simulink model "matlabVPC"  (R2021a)
settings: Solver=FixedStepAuto  StartTime=0.0  StopTime=tend  FixedStep=0.02  RelTol=1e-3
undefined symbols (not defined in the file): alpha, eta1, eta2, gd, Kc, offset1, offset2, pwo_init, scale1, scale2, T, v1, v2, var_max
libraries: simlib_vpc_basic x17, simlib_vpc_coremath x10, simlib_vpc_gp x3
settings Model: Creator=marco  LastModifiedBy=marco
settings DebuggingCC: AlgebraicLoopMsg=none  ArtificialAlgebraicLoopMsg=none

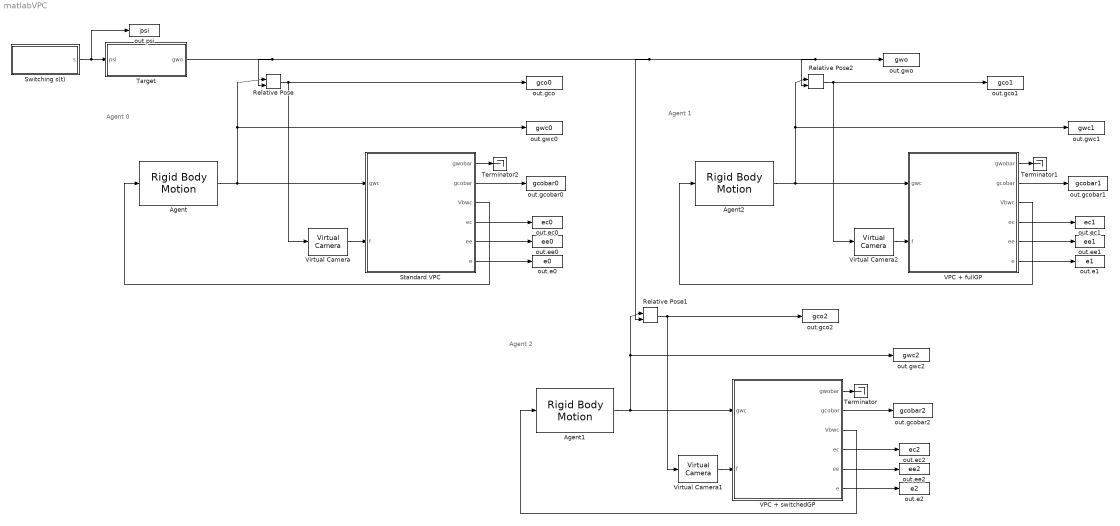
== system matlabVPC ==
  note: Agent 2
  note: Agent 1
  note: Agent 0
  Agent : simlib_vpc_basic/Rigid Body Motion  rbmtype=agent  agentnumber=1  projection=on  show_dg=off  g0=gwc_init
      settings: SourceProductName=VPC Library
  Agent1 : simlib_vpc_basic/Rigid Body Motion  rbmtype=agent  agentnumber=3  projection=on  show_dg=off  g0=gwc_init
      settings: SourceProductName=VPC Library
  Agent2 : simlib_vpc_basic/Rigid Body Motion  rbmtype=agent  agentnumber=2  projection=on  show_dg=off  g0=gwc_init
      settings: SourceProductName=VPC Library
  Relative Pose : simlib_vpc_coremath/Relative Pose
      settings: SourceProductName=VPC Library
  Relative Pose1 : simlib_vpc_coremath/Relative Pose
      settings: SourceProductName=VPC Library
  Relative Pose2 : simlib_vpc_coremath/Relative Pose
      settings: SourceProductName=VPC Library
  Standard VPC : Subsystem
      mask Display:
      | disp('VPC without GP','texmode','on')
      | 
      | % Label ports
      | port_label('input',1,'g_{wc}','texmode','on')
      | port_label('input',2,'f','texmode','on')
      | port_label('output',1,'g_{wo,bar}','texmode','on')
      | port_label('output',2,'gco,bar','texmode','on')
      | port_label('output',3,'V^b_{wc}','texmode','on')
      | port_label('output',4,'ec','texmode','on')
      | port_label('output',5,'ee','texmode','on')
      | port_label('output',6,'e','texmode','on')
  Switching s(t) : Subsystem
  Target : Subsystem
      mask Display:
      | % Glitch in Matlab: If you define a line whose starting point and end point
      | % is equal, then the entire mask block is plotted in bold
      | plot([0,0],[0,0])
      | 
      | % Draw Box
      | plot([0,1,1,0,0],[0,0,1,1,0])
      | 
      | % Write label
      | disp('Target','texmode','on')
      | 
      | % Image
      | p=get_param(gcb,'Position');
      | size = min(p(3:4)-p(1:2));
      | blkscale = abs((p(3)-p(1)) / (p(4)-p(2)));
      | if abs((p(3)-p(1))) > abs((p(4)-p(2))) % block is horizontal
      |     scale = .5*[1/blkscale .6];
      | else % block is vertical
      |     scale = .5*[1 .6*blkscale];
      | end
      | pos = [1-scale(1) 0.1]/2;
      | image('ico_target.png',[pos scale],'off')
      | 
      | % Label ports
      | port_label('output',1,['g_{wo}'],'texmode','on')
  Terminator : Terminator
  Terminator1 : Terminator
  Terminator2 : Terminator
  VPC + fullGP : Subsystem
      mask Display:
      | disp('VPC + fullGP','texmode','on')
      | 
      | % Label ports
      | port_label('input',1,'g_{wc}','texmode','on')
      | port_label('input',2,'f','texmode','on')
      | port_label('output',1,'g_{wo,bar}','texmode','on')
      | port_label('output',2,'gco,bar','texmode','on')
      | port_label('output',3,'V^b_{wc}','texmode','on')
      | port_label('output',4,'ec','texmode','on')
      | port_label('output',5,'ee','texmode','on')
      | port_label('output',6,'e','texmode','on')
  VPC + switchedGP : Subsystem
      mask Display:
      | disp('VPC + switchedGP','texmode','on')
      | 
      | % Label ports
      | port_label('input',1,'g_{wc}','texmode','on')
      | port_label('input',2,'f','texmode','on')
      | port_label('output',1,'g_{wo,bar}','texmode','on')
      | port_label('output',2,'gco,bar','texmode','on')
      | port_label('output',3,'V^b_{wc}','texmode','on')
      | port_label('output',4,'ec','texmode','on')
      | port_label('output',5,'ee','texmode','on')
      | port_label('output',6,'e','texmode','on')
  Virtual Camera : simlib_vpc_basic/Virtual Camera  camtype=Pinhole  po=fp  lambda=lambda
      settings: SourceProductName=VPC Library
  Virtual Camera1 : simlib_vpc_basic/Virtual Camera  camtype=Pinhole  po=fp  lambda=lambda
      settings: SourceProductName=VPC Library
  Virtual Camera2 : simlib_vpc_basic/Virtual Camera  camtype=Pinhole  po=fp  lambda=lambda
      settings: SourceProductName=VPC Library
  out.e0 : ToWorkspace  VariableName=e0  SaveFormat=Structure With Time  SampleTime=-1
  out.e1 : ToWorkspace  VariableName=e1  SaveFormat=Structure With Time  SampleTime=-1
  out.e2 : ToWorkspace  VariableName=e2  SaveFormat=Structure With Time  SampleTime=-1
  out.ec0 : ToWorkspace  VariableName=ec0  SaveFormat=Structure With Time  SampleTime=-1
  out.ec1 : ToWorkspace  VariableName=ec1  SaveFormat=Structure With Time  SampleTime=-1
  out.ec2 : ToWorkspace  VariableName=ec2  SaveFormat=Structure With Time  SampleTime=-1
  out.ee0 : ToWorkspace  VariableName=ee0  SaveFormat=Structure With Time  SampleTime=-1
  out.ee1 : ToWorkspace  VariableName=ee1  SaveFormat=Structure With Time  SampleTime=-1
  out.ee2 : ToWorkspace  VariableName=ee2  SaveFormat=Structure With Time  SampleTime=-1
  out.gco : ToWorkspace  VariableName=gco0  SaveFormat=Structure With Time  SampleTime=-1
  out.gco1 : ToWorkspace  VariableName=gco1  SaveFormat=Structure With Time  SampleTime=-1
  out.gco2 : ToWorkspace  VariableName=gco2  SaveFormat=Structure With Time  SampleTime=-1
  out.gcobar0 : ToWorkspace  VariableName=gcobar0  SaveFormat=Structure With Time  SampleTime=-1
  out.gcobar1 : ToWorkspace  VariableName=gcobar1  SaveFormat=Structure With Time  SampleTime=-1
  out.gcobar2 : ToWorkspace  VariableName=gcobar2  SaveFormat=Structure With Time  SampleTime=-1
  out.gwc0 : ToWorkspace  VariableName=gwc0  SaveFormat=Structure With Time  SampleTime=-1
  out.gwc1 : ToWorkspace  VariableName=gwc1  SaveFormat=Structure With Time  SampleTime=-1
  out.gwc2 : ToWorkspace  VariableName=gwc2  SaveFormat=Structure With Time  SampleTime=-1
  out.gwo : ToWorkspace  VariableName=gwo  SaveFormat=Structure With Time  SampleTime=-1
  out.psi : ToWorkspace  VariableName=psi  SaveFormat=Structure With Time  SampleTime=-1
  wires:
  Relative Pose2/1 -> Virtual Camera2/1, out.gco1/1
  Relative Pose/1 -> Virtual Camera/1, out.gco/1
  VPC + fullGP/2(gcobar) -> out.gcobar1/1
  VPC + switchedGP/4(ec) -> out.ec2/1
  Relative Pose1/1 -> Virtual Camera1/1, out.gco2/1
  Agent1/1 -> VPC + switchedGP/1(gwc), out.gwc2/1, Relative Pose1/1
  Switching s(t)/1(s) -> out.psi/1, Target/1(psi)
  Virtual Camera/1 -> Standard VPC/2(f)
  VPC + switchedGP/2(gcobar) -> out.gcobar2/1
  Virtual Camera2/1 -> VPC + fullGP/2(f)
  VPC + switchedGP/5(ee) -> out.ee2/1
  VPC + fullGP/4(ec) -> out.ec1/1
  VPC + switchedGP/6(e) -> out.e2/1
  Virtual Camera1/1 -> VPC + switchedGP/2(f)
  Agent/1 -> Standard VPC/1(gwc), out.gwc0/1, Relative Pose/1
  Standard VPC/6(e) -> out.e0/1
  Target/1(gwo) -> Relative Pose2/2, out.gwo/1, Relative Pose1/2, Relative Pose/2
  Standard VPC/4(ec) -> out.ec0/1
  Standard VPC/5(ee) -> out.ee0/1
  Agent2/1 -> VPC + fullGP/1(gwc), out.gwc1/1, Relative Pose2/1
  Standard VPC/2(gcobar) -> out.gcobar0/1
  VPC + fullGP/5(ee) -> out.ee1/1
  VPC + fullGP/6(e) -> out.e1/1
  Standard VPC/3(Vbwc) -> Agent/1
  VPC + switchedGP/3(Vbwc) -> Agent1/1
  VPC + fullGP/3(Vbwc) -> Agent2/1
  VPC + switchedGP/1(gwobar) -> Terminator/1
  VPC + fullGP/1(gwobar) -> Terminator1/1
  Standard VPC/1(gwobar) -> Terminator2/1

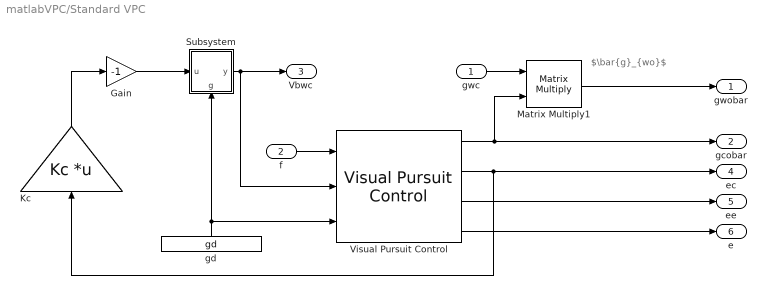
== system matlabVPC/Standard VPC ==
  note: $\bar{g}_{wo}$
  gwc : Inport
  f : Inport  Port=2
  Gain : Gain  Gain=-1
  Kc : Gain  Gain=Kc  Multiplication=Matrix(K*u) (u vector)
  Matrix Multiply1 : Product  Multiplication=Matrix(*)
  Subsystem : Subsystem
      settings: PortSchema="{\"entries\":[{\"content\":{\"sides\":[{\"content\":{\"connectorIds\":[\"In1\"]},\"type\":\"ConnectorPlacement.EquallySpacedRectSide\",\"uuid\":\"72e68008-5c4a-43a9-a560-64c6a31a0c08\"},{\"content\":{\"connectorIds\":[\"Out1\"],\"side\":\"RIGHT\"},\"type\":\"ConnectorPlacement.EquallySpacedRectSide\",\"uuid\":\"da07f5ff-2b2c-4c55-a2f2-34e133777503\"},{\"content\":{\"connectorIds\":[],\"side\":\"TOP\"},\"type\":\"ConnectorPlacement.EquallySpacedRectSide\",\"uuid\":\"6d174428-4364-4e89-aba7-4e9864808ab5\"},{\"content\":{\"connectorIds\":[\"In2\"],\"side\":\"BOTTOM\"},\"type\":\"ConnectorPlacement.EquallySpacedRectSide\",\"uuid\":\"f9633104-9c11-4d21-90a7-e0f886d9e92d\"},{\"content\":{\"connectorIds\":[],\"side\":\"HIDDEN\"},\"type\":\"ConnectorPlacement.EquallySpacedRectSide\",\"uuid\":\"662f08ae-9279-4a4f-85ea-81d97ead27d9\"}]},\"type\":\"ConnectorPlacement.EquallySpacedConnector\",\"uuid\":\"f3cd156c-cccd-47c6-b81c-6113f78efd58\"}],\"packageUris\":[\"http://schema.mathworks.com/mf0/Connector/R2020b\"],\"version\":\"1.0\"}"
      mask Display:
      | % Glitch in Matlab: If you define a line whose starting point and end point
      | % is equal, then the entire mask block is plotted in bold
      | plot([0,0],[0,0])
      | 
      | % Draw box
      | indent = 0.3;
      | ang=[0:0.2:pi/2, pi/2];
      | plot([0,1-indent],[0,0])
      | xp=indent*sin(ang)+1-indent;
      | yp=indent-indent*cos(ang);
      | plot(xp,yp);
      | plot([1,1,indent],[indent,1,1])
      | xp=indent-indent*sin(ang);
      | yp=1-indent+indent*cos(ang);
      | plot(xp,yp);
      | plot([0,0],[1-indent,0])
      | 
      | % Write label & ports
      | disp('-Ad_{(g_d)}','texmode','on')
      | text(0.5,0.2,'\fontsize{7}g_d','texmode','on')
  Visual Pursuit Control : simlib_vpc_basic/Visual Pursuit Control  gd_source=external  gd_value=[eye(4,3),ones(4,1)]  show_ee=on  show_e=on  show_nu=off  show_dgcobar=off  show_gce=off  gcobar0=gco_init  Ke_source=internal  Ke=Ke  show_ue_aux=off  projection=on  camtype=Pinhole  fo=fp  lambda=lambda
      settings: SourceProductName=VPC Library
  gd : Constant  Value=gd
  gwobar : Outport
  gcobar : Outport  Port=2
  Vbwc : Outport  Port=3
  ec : Outport  Port=4
  ee : Outport  Port=5
  e : Outport  Port=6
  wires:
  f/1 -> Visual Pursuit Control/1
  Matrix Multiply1/1 -> gwobar/1
  Subsystem/1(y) -> Vbwc/1, Visual Pursuit Control/2
  gwc/1 -> Matrix Multiply1/1
  Kc/1 -> Gain/1
  Visual Pursuit Control/4 -> e/1
  Gain/1 -> Subsystem/1(u)
  Visual Pursuit Control/2 -> ec/1, Kc/1
  Visual Pursuit Control/3 -> ee/1
  gd/1 -> Subsystem/2(g), Visual Pursuit Control/3
  Visual Pursuit Control/1 -> gcobar/1, Matrix Multiply1/2

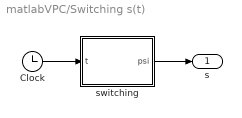
== system matlabVPC/Switching s(t) ==
  Clock : Clock
  switching : MATLAB Function  TreatAsAtomicUnit=on
  s : Outport
  wires:
  Clock/1 -> switching/1(t)
  switching/1(psi) -> s/1

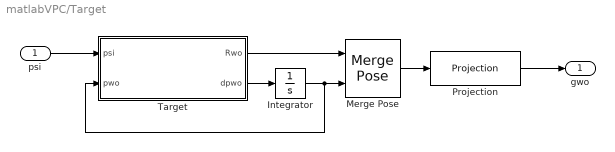
== system matlabVPC/Target ==
  psi : Inport
  Integrator : Integrator  InitialCondition=pwo_init  ContinuousStateAttributes='pose'
  Merge Pose : simlib_vpc_coremath/Merge Pose
      settings: SourceProductName=VPC Library
  Projection : simlib_vpc_basic/Projection  projectiontype=averaging  inputtype=pose
      settings: SourceProductName=VPC Library
  Target : MATLAB Function  TreatAsAtomicUnit=on
  gwo : Outport
  wires:
  Merge Pose/1 -> Projection/1
  Projection/1 -> gwo/1
  Integrator/1 -> Target/2(pwo), Merge Pose/2
  Target/2(dpwo) -> Integrator/1
  Target/1(Rwo) -> Merge Pose/1
  psi/1 -> Target/1(psi)

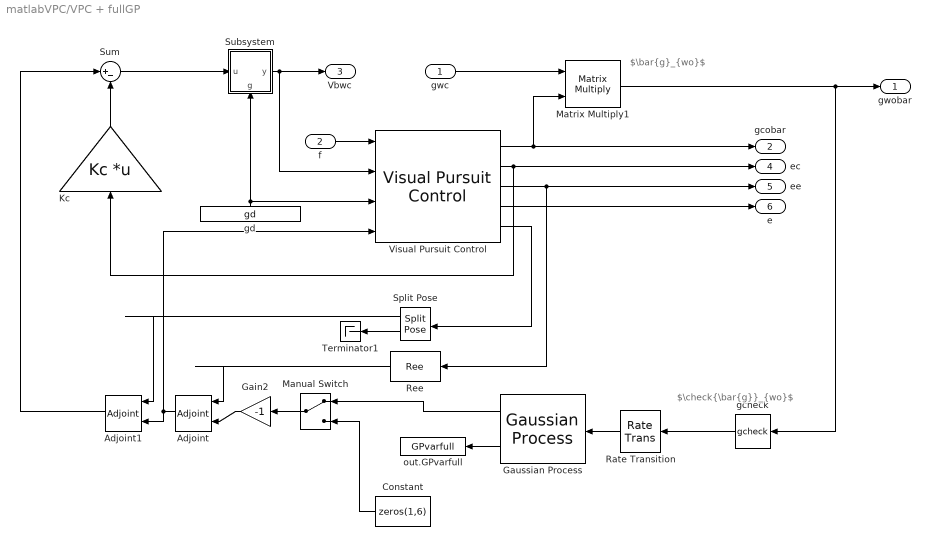
== system matlabVPC/VPC + fullGP ==
  note: $\bar{g}_{wo}$
  note: $\check{\bar{g}}_{wo}$
  gwc : Inport
  f : Inport  Port=2
  Adjoint : simlib_vpc_basic/Adjoint  adjointtype=orientation
      settings: SourceProductName=VPC Library
  Adjoint1 : simlib_vpc_basic/Adjoint  adjointtype=orientation
      settings: SourceProductName=VPC Library
  Constant : Constant  Value=zeros(1,6)
  Gain2 : Gain  Gain=-1
  Gaussian Process : simlib_vpc_gp/Gaussian Process  X=Xfull  Y=Yfull  sigman=snfull  kernel=Squared Exponential ARD  hyp=hypfull
      settings: SourceProductName=VPC Library
  Kc : Gain  Gain=Kc  Multiplication=Matrix(K*u) (u vector)
  Manual Switch : ManualSwitch
  Matrix Multiply1 : Product  Multiplication=Matrix(*)
  Rate Transition : RateTransition
  Ree : simlib_vpc_coremath/Ree
      settings: SourceProductName=VPC Library
  Split Pose : simlib_vpc_coremath/Split Pose
      settings: SourceProductName=VPC Library
  Subsystem : Subsystem
      settings: PortSchema="{\"entries\":[{\"content\":{\"sides\":[{\"content\":{\"connectorIds\":[\"In1\"]},\"type\":\"ConnectorPlacement.EquallySpacedRectSide\",\"uuid\":\"72e68008-5c4a-43a9-a560-64c6a31a0c08\"},{\"content\":{\"connectorIds\":[\"Out1\"],\"side\":\"RIGHT\"},\"type\":\"ConnectorPlacement.EquallySpacedRectSide\",\"uuid\":\"da07f5ff-2b2c-4c55-a2f2-34e133777503\"},{\"content\":{\"connectorIds\":[],\"side\":\"TOP\"},\"type\":\"ConnectorPlacement.EquallySpacedRectSide\",\"uuid\":\"6d174428-4364-4e89-aba7-4e9864808ab5\"},{\"content\":{\"connectorIds\":[\"In2\"],\"side\":\"BOTTOM\"},\"type\":\"ConnectorPlacement.EquallySpacedRectSide\",\"uuid\":\"f9633104-9c11-4d21-90a7-e0f886d9e92d\"},{\"content\":{\"connectorIds\":[],\"side\":\"HIDDEN\"},\"type\":\"ConnectorPlacement.EquallySpacedRectSide\",\"uuid\":\"662f08ae-9279-4a4f-85ea-81d97ead27d9\"}]},\"type\":\"ConnectorPlacement.EquallySpacedConnector\",\"uuid\":\"f3cd156c-cccd-47c6-b81c-6113f78efd58\"}],\"packageUris\":[\"http://schema.mathworks.com/mf0/Connector/R2020b\"],\"version\":\"1.0\"}"
      mask Display:
      | % Glitch in Matlab: If you define a line whose starting point and end point
      | % is equal, then the entire mask block is plotted in bold
      | plot([0,0],[0,0])
      | 
      | % Draw box
      | indent = 0.3;
      | ang=[0:0.2:pi/2, pi/2];
      | plot([0,1-indent],[0,0])
      | xp=indent*sin(ang)+1-indent;
      | yp=indent-indent*cos(ang);
      | plot(xp,yp);
      | plot([1,1,indent],[indent,1,1])
      | xp=indent-indent*sin(ang);
      | yp=1-indent+indent*cos(ang);
      | plot(xp,yp);
      | plot([0,0],[1-indent,0])
      | 
      | % Write label & ports
      | disp('-Ad_{(g_d)}','texmode','on')
      | text(0.5,0.2,'\fontsize{7}g_d','texmode','on')
  Sum : Sum  Inputs=|+-
  Terminator1 : Terminator
  Visual Pursuit Control : simlib_vpc_basic/Visual Pursuit Control  gd_source=external  gd_value=[eye(4,3),ones(4,1)]  show_ee=on  show_e=on  show_nu=off  show_dgcobar=off  show_gce=on  gcobar0=gco_init  Ke_source=internal  Ke=Ke  show_ue_aux=on  projection=on  camtype=Pinhole  fo=fp  lambda=lambda
      settings: SourceProductName=VPC Library
  gcheck : simlib_vpc_coremath/gcheck
      settings: SourceProductName=VPC Library
  gd : Constant  Value=gd
  out.GPvarfull : ToWorkspace  VariableName=GPvarfull  SaveFormat=Structure With Time  SampleTime=-1
  gwobar : Outport
  gcobar : Outport  Port=2
  Vbwc : Outport  Port=3
  ec : Outport  Port=4
  ee : Outport  Port=5
  e : Outport  Port=6
  wires:
  f/1 -> Visual Pursuit Control/1
  Matrix Multiply1/1 -> gcheck/1, gwobar/1
  Subsystem/1(y) -> Vbwc/1, Visual Pursuit Control/2
  gwc/1 -> Matrix Multiply1/1
  Visual Pursuit Control/4 -> e/1
  Kc/1 -> Sum/2
  Visual Pursuit Control/2 -> ec/1, Kc/1
  Visual Pursuit Control/3 -> Ree/1, ee/1
  gd/1 -> Subsystem/2(g), Visual Pursuit Control/3
  Visual Pursuit Control/1 -> Matrix Multiply1/2, gcobar/1
  Split Pose/1 -> Adjoint1/2
  Rate Transition/1 -> Gaussian Process/1
  Adjoint/1 -> Visual Pursuit Control/4, Adjoint1/1
  Ree/1 -> Adjoint/2
  Split Pose/2 -> Terminator1/1
  Gain2/1 -> Adjoint/1
  Manual Switch/1 -> Gain2/1
  Sum/1 -> Subsystem/1(u)
  Adjoint1/1 -> Sum/1
  Visual Pursuit Control/5 -> Split Pose/1
  Gaussian Process/2 -> out.GPvarfull/1
  gcheck/1 -> Rate Transition/1
  Gaussian Process/1 -> Manual Switch/1
  Constant/1 -> Manual Switch/2

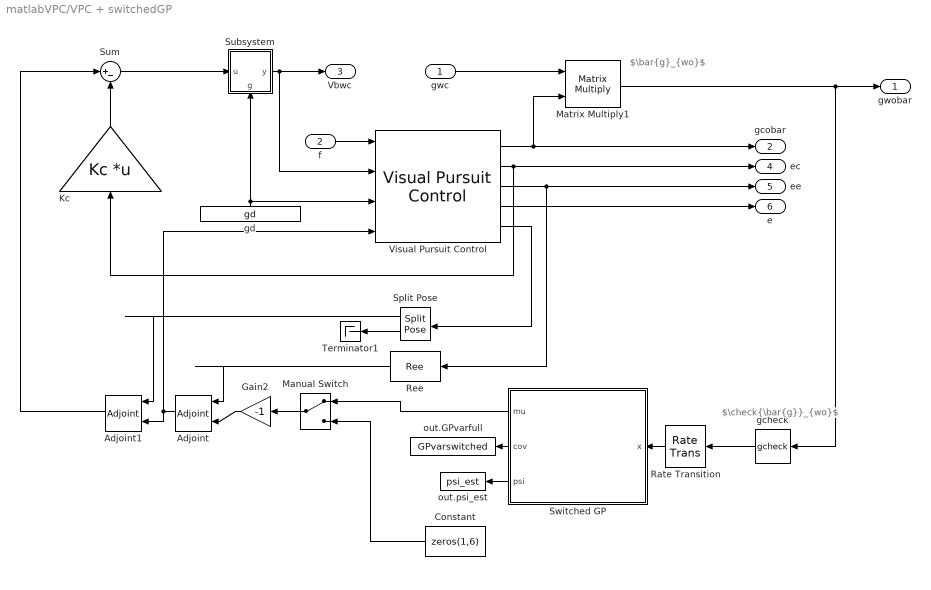
== system matlabVPC/VPC + switchedGP ==
  note: $\bar{g}_{wo}$
  note: $\check{\bar{g}}_{wo}$
  gwc : Inport
  f : Inport  Port=2
  Adjoint : simlib_vpc_basic/Adjoint  adjointtype=orientation
      settings: SourceProductName=VPC Library
  Adjoint1 : simlib_vpc_basic/Adjoint  adjointtype=orientation
      settings: SourceProductName=VPC Library
  Constant : Constant  Value=zeros(1,6)
  Gain2 : Gain  Gain=-1
  Kc : Gain  Gain=Kc  Multiplication=Matrix(K*u) (u vector)
  Manual Switch : ManualSwitch
  Matrix Multiply1 : Product  Multiplication=Matrix(*)
  Rate Transition : RateTransition
  Ree : simlib_vpc_coremath/Ree
      settings: SourceProductName=VPC Library
  Split Pose : simlib_vpc_coremath/Split Pose
      settings: SourceProductName=VPC Library
  Subsystem : Subsystem
      settings: PortSchema="{\"entries\":[{\"content\":{\"sides\":[{\"content\":{\"connectorIds\":[\"In1\"]},\"type\":\"ConnectorPlacement.EquallySpacedRectSide\",\"uuid\":\"72e68008-5c4a-43a9-a560-64c6a31a0c08\"},{\"content\":{\"connectorIds\":[\"Out1\"],\"side\":\"RIGHT\"},\"type\":\"ConnectorPlacement.EquallySpacedRectSide\",\"uuid\":\"da07f5ff-2b2c-4c55-a2f2-34e133777503\"},{\"content\":{\"connectorIds\":[],\"side\":\"TOP\"},\"type\":\"ConnectorPlacement.EquallySpacedRectSide\",\"uuid\":\"6d174428-4364-4e89-aba7-4e9864808ab5\"},{\"content\":{\"connectorIds\":[\"In2\"],\"side\":\"BOTTOM\"},\"type\":\"ConnectorPlacement.EquallySpacedRectSide\",\"uuid\":\"f9633104-9c11-4d21-90a7-e0f886d9e92d\"},{\"content\":{\"connectorIds\":[],\"side\":\"HIDDEN\"},\"type\":\"ConnectorPlacement.EquallySpacedRectSide\",\"uuid\":\"662f08ae-9279-4a4f-85ea-81d97ead27d9\"}]},\"type\":\"ConnectorPlacement.EquallySpacedConnector\",\"uuid\":\"f3cd156c-cccd-47c6-b81c-6113f78efd58\"}],\"packageUris\":[\"http://schema.mathworks.com/mf0/Connector/R2020b\"],\"version\":\"1.0\"}"
      mask Display:
      | % Glitch in Matlab: If you define a line whose starting point and end point
      | % is equal, then the entire mask block is plotted in bold
      | plot([0,0],[0,0])
      | 
      | % Draw box
      | indent = 0.3;
      | ang=[0:0.2:pi/2, pi/2];
      | plot([0,1-indent],[0,0])
      | xp=indent*sin(ang)+1-indent;
      | yp=indent-indent*cos(ang);
      | plot(xp,yp);
      | plot([1,1,indent],[indent,1,1])
      | xp=indent-indent*sin(ang);
      | yp=1-indent+indent*cos(ang);
      | plot(xp,yp);
      | plot([0,0],[1-indent,0])
      | 
      | % Write label & ports
      | disp('-Ad_{(g_d)}','texmode','on')
      | text(0.5,0.2,'\fontsize{7}g_d','texmode','on')
  Sum : Sum  Inputs=|+-
  Switched GP : Subsystem
      mask Display:
      | disp('Switched GP','texmode','on')
      | 
      | % Label ports
      | port_label('input',1,'x*','texmode','on')
      | port_label('output',1,'\mu','texmode','on')
      | port_label('output',2,'\Sigma','texmode','on')
      | port_label('output',3,'\psi_{est}','texmode','on')
  Terminator1 : Terminator
  Visual Pursuit Control : simlib_vpc_basic/Visual Pursuit Control  gd_source=external  gd_value=[eye(4,3),ones(4,1)]  show_ee=on  show_e=on  show_nu=off  show_dgcobar=off  show_gce=on  gcobar0=gco_init  Ke_source=internal  Ke=Ke  show_ue_aux=on  projection=on  camtype=Pinhole  fo=fp  lambda=lambda
      settings: SourceProductName=VPC Library
  gcheck : simlib_vpc_coremath/gcheck
      settings: SourceProductName=VPC Library
  gd : Constant  Value=gd
  out.GPvarfull : ToWorkspace  VariableName=GPvarswitched  SaveFormat=Structure With Time  SampleTime=-1
  out.psi_est : ToWorkspace  VariableName=psi_est  SaveFormat=Structure With Time  SampleTime=-1
  gwobar : Outport
  gcobar : Outport  Port=2
  Vbwc : Outport  Port=3
  ec : Outport  Port=4
  ee : Outport  Port=5
  e : Outport  Port=6
  wires:
  f/1 -> Visual Pursuit Control/1
  Matrix Multiply1/1 -> gcheck/1, gwobar/1
  Subsystem/1(y) -> Vbwc/1, Visual Pursuit Control/2
  gwc/1 -> Matrix Multiply1/1
  Visual Pursuit Control/4 -> e/1
  Kc/1 -> Sum/2
  Visual Pursuit Control/2 -> ec/1, Kc/1
  Visual Pursuit Control/3 -> Ree/1, ee/1
  gd/1 -> Subsystem/2(g), Visual Pursuit Control/3
  Visual Pursuit Control/1 -> Matrix Multiply1/2, gcobar/1
  Split Pose/1 -> Adjoint1/2
  Adjoint/1 -> Visual Pursuit Control/4, Adjoint1/1
  Ree/1 -> Adjoint/2
  Split Pose/2 -> Terminator1/1
  Gain2/1 -> Adjoint/1
  Sum/1 -> Subsystem/1(u)
  Adjoint1/1 -> Sum/1
  Visual Pursuit Control/5 -> Split Pose/1
  gcheck/1 -> Rate Transition/1
  Switched GP/3(psi) -> out.psi_est/1
  Rate Transition/1 -> Switched GP/1(x)
  Switched GP/2(cov) -> out.GPvarfull/1
  Switched GP/1(mu) -> Manual Switch/1
  Manual Switch/1 -> Gain2/1
  Constant/1 -> Manual Switch/2

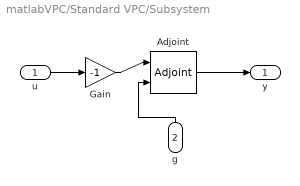
== system matlabVPC/Standard VPC/Subsystem ==
  u : Inport
  g : Inport  Port=2
  Adjoint : simlib_vpc_basic/Adjoint  adjointtype=pose
      settings: SourceProductName=VPC Library
  Gain : Gain  Gain=-1
  y : Outport
  wires:
  Adjoint/1 -> y/1
  u/1 -> Gain/1
  g/1 -> Adjoint/2
  Gain/1 -> Adjoint/1

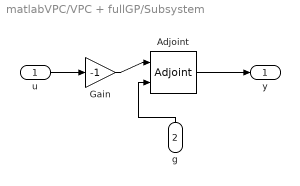
== system matlabVPC/VPC + fullGP/Subsystem ==
  u : Inport
  g : Inport  Port=2
  Adjoint : simlib_vpc_basic/Adjoint  adjointtype=pose
      settings: SourceProductName=VPC Library
  Gain : Gain  Gain=-1
  y : Outport
  wires:
  Adjoint/1 -> y/1
  u/1 -> Gain/1
  g/1 -> Adjoint/2
  Gain/1 -> Adjoint/1

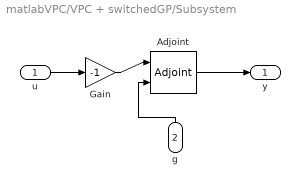
== system matlabVPC/VPC + switchedGP/Subsystem ==
  u : Inport
  g : Inport  Port=2
  Adjoint : simlib_vpc_basic/Adjoint  adjointtype=pose
      settings: SourceProductName=VPC Library
  Gain : Gain  Gain=-1
  y : Outport
  wires:
  Adjoint/1 -> y/1
  u/1 -> Gain/1
  g/1 -> Adjoint/2
  Gain/1 -> Adjoint/1

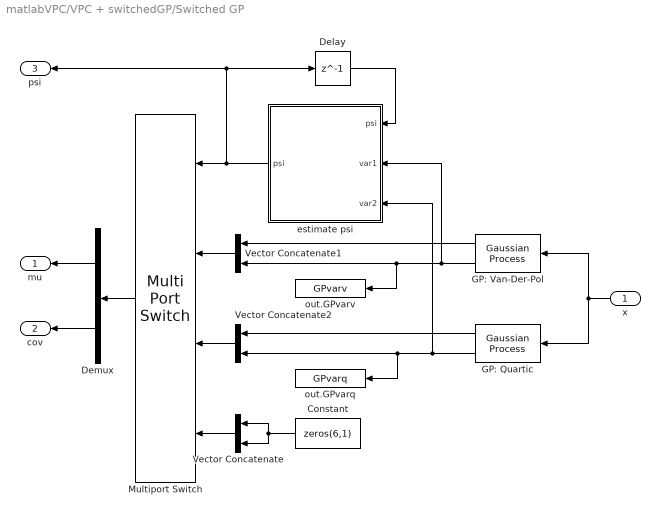
== system matlabVPC/VPC + switchedGP/Switched GP ==
  x : Inport
  Constant : Constant  Value=zeros(6,1)
  Delay : Delay  DelayLength=1
  Demux : Demux  Outputs=2
  GP: Quartic : simlib_vpc_gp/Gaussian Process  X=X2  Y=Y2  sigman=sn2  kernel=Squared Exponential ARD  hyp=hyp2
      settings: SourceProductName=VPC Library
  GP: Van-Der-Pol : simlib_vpc_gp/Gaussian Process  X=X1  Y=Y1  sigman=sn1  kernel=Squared Exponential ARD  hyp=hyp1
      settings: SourceProductName=VPC Library
  Multiport Switch : MultiPortSwitch  Inputs=2  DataPortForDefault=Additional data port
  Vector Concatenate : Concatenate
  Vector Concatenate1 : Concatenate
  Vector Concatenate2 : Concatenate
  estimate psi : MATLAB Function  TreatAsAtomicUnit=on
  out.GPvarq : ToWorkspace  VariableName=GPvarq  SaveFormat=Structure With Time  SampleTime=-1
  out.GPvarv : ToWorkspace  VariableName=GPvarv  SaveFormat=Structure With Time  SampleTime=-1
  mu : Outport
  cov : Outport  Port=2
  psi : Outport  Port=3
  wires:
  Constant/1 -> Vector Concatenate/2, Vector Concatenate/1
  Vector Concatenate/1 -> Multiport Switch/4
  Vector Concatenate1/1 -> Multiport Switch/2
  Multiport Switch/1 -> Demux/1
  Vector Concatenate2/1 -> Multiport Switch/3
  GP: Quartic/1 -> Vector Concatenate2/1
  GP: Van-Der-Pol/1 -> Vector Concatenate1/1
  GP: Quartic/2 -> estimate psi/3(var2), out.GPvarq/1, Vector Concatenate2/2
  GP: Van-Der-Pol/2 -> estimate psi/2(var1), out.GPvarv/1, Vector Concatenate1/2
  Demux/1 -> mu/1
  Demux/2 -> cov/1
  x/1 -> GP: Quartic/1, GP: Van-Der-Pol/1
  estimate psi/1(psi) -> psi/1, Delay/1, Multiport Switch/1
  Delay/1 -> estimate psi/1("psi ")

== matlab function matlabVPC/VPC + switchedGP/Switched GP/estimate psi ==
  data: psi input; var1 input; psi output; var2 input; var_max parameter; T parameter; alpha parameter
function psi = estim_psi(psi,var1,var2,var_max,T, alpha)
%%ESTIM_PSI estimates the switching signal s(t)
%
% Editor:
%   OMAINSKA Marco - Doctoral Student, Cybernetics
%       <marcoomainska@g.ecc.u-tokyo.ac.jp>
% Review:
%   YAMAUCHI Junya - Assistant Professor
%       <junya_yamauchi@ipc.i.u-tokyo.ac.jp>
%
% Property of: Fujita-Yamauchi Lab, University of Tokyo, 2021
% e-mail: marcoomainska@g.ecc.u-tokyo.ac.jp
% Website: https://www.scl.ipc.i.u-tokyo.ac.jp
% February 2022
%
%------------- BEGIN CODE --------------

% calculate norms
var_norm = zeros(2,1);
var_norm(1) = norm(dot(alpha,var1),2)/var_max(1);
var_norm(2) = norm(dot(alpha,var2),2)/var_max(2);

% estimate switching
if psi == 0 % init case: psi is zero
    [~,psi] = min(var_norm); % find the smallest ||var||/var_max
else
    [~,psi_new] = min(var_norm); % find the smallest ||var||/var_max
    if var_norm(psi) > var_norm(psi_new) + T
        psi = psi_new;
    end
end

% fail safe case
if isnan(psi)
    psi = 0;
end

%-------------- END CODE ---------------
end

== matlab function matlabVPC/Switching s(t)/switching ==
  data: t input; psi output
function psi = s(t)

psi = 0;
if t < 4.5
    psi = 2;
elseif t < 8
    psi = 1;
elseif t < 20
    psi = 2;
else
    psi = 1;
end

end

== matlab function matlabVPC/Target/Target ==
  data: psi input; pwo input; eta1 parameter; eta2 parameter; v1 parameter; v2 parameter; scale1 parameter; Rwo output; dpwo output; scale2 parameter; offset1 parameter; offset2 parameter
function [Rwo, dpwo] = target_trajectory(psi, pwo, eta1, eta2, v1, v2, scale1, scale2, offset1, offset2) %#codegen
% Target Movement, Van-Der-Pol
%
% Editor:
%   OMAINSKA Marco - Doctoral Student, Cybernetics
%       <marcoomainska@g.ecc.u-tokyo.ac.jp>
% Review:
%   YAMAUCHI Junya - Assistant Professor
%       <junya_yamauchi@ipc.i.u-tokyo.ac.jp>
%
% Property of: Fujita-Yamauchi Lab, University of Tokyo, 2022
% e-mail: marcoomainska@g.ecc.u-tokyo.ac.jp
% Website: https://www.scl.ipc.i.u-tokyo.ac.jp
% March 2022
%
%------------- BEGIN CODE --------------

% Get velocity
switch psi
    case 1 % vanderpol 1st
        dpwo = v1 .* vanderpol((pwo(:) - offset1(:)) ./ scale1, eta1);
    case 2 % vanderpol 2nd
        dpwo = v2 .* vanderpol((pwo(:) - offset2(:)) ./ scale2, eta2);
    otherwise % vanderpol
        dpwo = v1 .* vanderpol((pwo(:) - offset1(:)) ./ scale1, eta1);
end

% set heading angle
angle = rad2deg(atan2(dpwo(2),dpwo(1)) - pi/2);
Rwo = rotz(angle);

%------------- END CODE --------------
end

function dpwo = vanderpol(pwo, epsilon)
% Van-Der-Pol trajectory
%
% Editor:
%   OMAINSKA Marco - Doctoral Student, Cybernetics
%       <marcoomainska@g.ecc.u-tokyo.ac.jp>
% Review:
%   YAMAUCHI Junya - Assistant Professor
%       <junya_yamauchi@ipc.i.u-tokyo.ac.jp>
%
% Property of: Fujita-Yamauchi Lab, University of Tokyo, 2022
% e-mail: marcoomainska@g.ecc.u-tokyo.ac.jp
% Website: https://www.scl.ipc.i.u-tokyo.ac.jp
% March 2022
%
%------------- BEGIN CODE --------------

dpwo = zeros(1,3);
dpwo(1) = pwo(2);
dpwo(2) = -pwo(1) + epsilon * (1 - pwo(1)^2) * pwo(2);

%------------- END CODE --------------
end
